simulink model "DCMotorControl_PI"  (R2024b)
settings: Solver=VariableStepAuto  StartTime=0.0  StopTime=0.2  RelTol=1e-4
InitFcn:
  | clear
  | clc
  | 
  | Power = 3336;
  | Vdc = 140;
  | Va_rated = 140;
  | Ia_rated = 25;
  | Wm_rated = 3000*2*pi/60;
  | Te_rated = Power/Wm_rated;
  | 
  | Ra = 0.26;
  | La = 1.7e-3;
  | J = 0.00252;
  | B = 0;
  | 
  | K = Te_rated/Ia_rated;
  | 
  | Wcc=500*2*pi;
  | Wcs=30*2*pi;
  | 
  | Kpc=La*Wcc;
  | Kic=Ra*Wcc;
  | Kac=1/Kpc;
  | 
  | Kps=(J*Wcs)/K;
  | Kis=(J*(Wcs)^2)/5*K;
  | Kas=1/Kps;
libraries: simulink x2
settings Model: Creator=junheehan  LastModifiedBy=junheehan

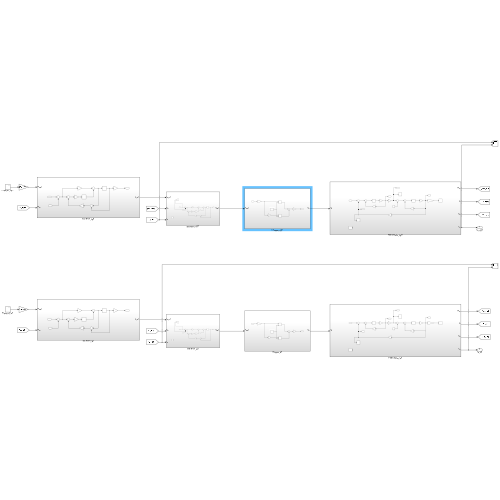
[thumbnail: Simulink's stored preview of the top-level diagram]
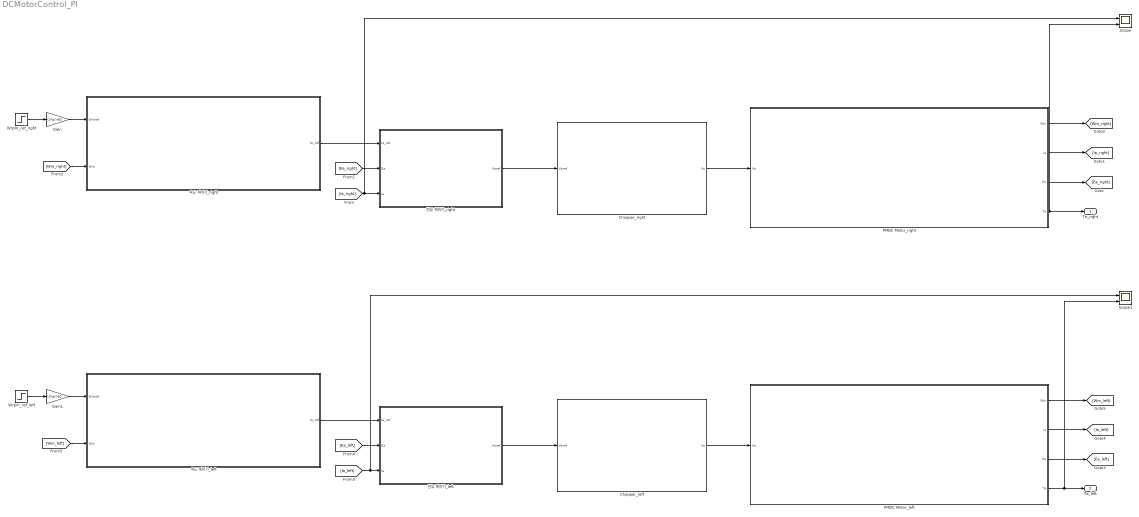
== system DCMotorControl_PI ==
  Chopper_left : Subsystem
  Chopper_right : Subsystem
  Gain : Gain  Gain=(2*pi)/60
  Gain1 : Gain  Gain=(2*pi)/60
  PMDC Motor_left : Subsystem
  PMDC Motor_right : Subsystem
  Scope : Scope  NumInputPorts=2
  Scope1 : Scope  NumInputPorts=2
  Wrpm_ref_left : Step  Time=0.05  After=2500  SampleTime=0
  Wrpm_ref_right : Step  Time=0.05  After=2500  SampleTime=0
  속도 제어기_left : Subsystem
  속도 제어기_right : Subsystem
  전류 제어기_left : Subsystem
  전류 제어기_right : Subsystem
  Te_right : Outport
  Te_left : Outport  Port=2
  wires:
  [Ea_right] -> 전류 제어기_right/2(Ea)
  [Ia_right] -> Scope/1, 전류 제어기_right/3(Ia)
  [Wm_right] -> 속도 제어기_right/2(Wm)
  속도 제어기_right/1(Ia_ref) -> 전류 제어기_right/1(Ia_ref)
  PMDC Motor_right/1(Wm) -> [Wm_right]
  PMDC Motor_right/3(Ea) -> [Ea_right]
  PMDC Motor_right/2(Ia) -> [Ia_right]
  Wrpm_ref_right/1 -> Gain/1
  Gain/1 -> 속도 제어기_right/1(Wmref)
  전류 제어기_right/1(Varef) -> Chopper_right/1(Varef)
  Chopper_right/1(Va) -> PMDC Motor_right/1(Va)
  PMDC Motor_right/4(Te) -> Scope/2, Te_right/1
  [Ea_left] -> 전류 제어기_left/2(Ea)
  전류 제어기_left/1(Varef) -> Chopper_left/1(Varef)
  PMDC Motor_left/1(Wm) -> [Wm_left]
  Gain1/1 -> 속도 제어기_left/1(Wmref)
  PMDC Motor_left/4(Te) -> Scope1/2, Te_left/1
  PMDC Motor_left/2(Ia) -> [Ia_left]
  Wrpm_ref_left/1 -> Gain1/1
  Chopper_left/1(Va) -> PMDC Motor_left/1(Va)
  [Ia_left] -> Scope1/1, 전류 제어기_left/3(Ia)
  [Wm_left] -> 속도 제어기_left/2(Wm)
  속도 제어기_left/1(Ia_ref) -> 전류 제어기_left/1(Ia_ref)
  PMDC Motor_left/3(Ea) -> [Ea_left]

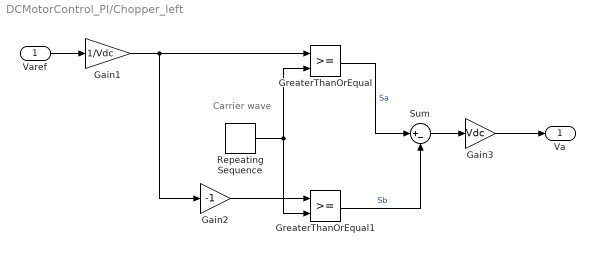
== system DCMotorControl_PI/Chopper_left ==
  note: Carrier wave
  Varef : Inport
  Gain1 : Gain  Gain=1/Vdc
  Gain2 : Gain  Gain=-1
  Gain3 : Gain  Gain=Vdc
  GreaterThanOrEqual : RelationalOperator  OutDataTypeStr=boolean  RndMeth=Simplest  InputSameDT=off
  GreaterThanOrEqual1 : RelationalOperator  OutDataTypeStr=boolean  RndMeth=Simplest  InputSameDT=off
  Repeating Sequence : simulink/Sources/Repeating Sequence  rep_seq_t=[0 1/10000 1/5000]  rep_seq_y=[-1 1 -1]
  Sum : Sum  Inputs=|+-
  Va : Outport
  wires:
  Varef/1 -> Gain1/1
  GreaterThanOrEqual1/1 -> Sum/2  "Sb"
  GreaterThanOrEqual/1 -> Sum/1  "Sa"
  Gain3/1 -> Va/1
  Repeating Sequence/1 -> GreaterThanOrEqual1/2, GreaterThanOrEqual/2
  Gain2/1 -> GreaterThanOrEqual1/1
  Gain1/1 -> Gain2/1, GreaterThanOrEqual/1
  Sum/1 -> Gain3/1

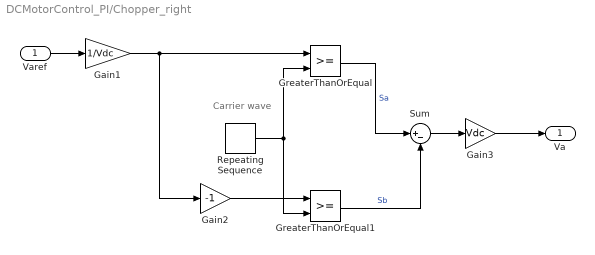
== system DCMotorControl_PI/Chopper_right ==
  note: Carrier wave
  Varef : Inport
  Gain1 : Gain  Gain=1/Vdc
  Gain2 : Gain  Gain=-1
  Gain3 : Gain  Gain=Vdc
  GreaterThanOrEqual : RelationalOperator  OutDataTypeStr=boolean  RndMeth=Simplest  InputSameDT=off
  GreaterThanOrEqual1 : RelationalOperator  OutDataTypeStr=boolean  RndMeth=Simplest  InputSameDT=off
  Repeating Sequence : simulink/Sources/Repeating Sequence  rep_seq_t=[0 1/10000 1/5000]  rep_seq_y=[-1 1 -1]
  Sum : Sum  Inputs=|+-
  Va : Outport
  wires:
  Varef/1 -> Gain1/1
  GreaterThanOrEqual1/1 -> Sum/2  "Sb"
  GreaterThanOrEqual/1 -> Sum/1  "Sa"
  Gain3/1 -> Va/1
  Repeating Sequence/1 -> GreaterThanOrEqual1/2, GreaterThanOrEqual/2
  Gain2/1 -> GreaterThanOrEqual1/1
  Gain1/1 -> Gain2/1, GreaterThanOrEqual/1
  Sum/1 -> Gain3/1

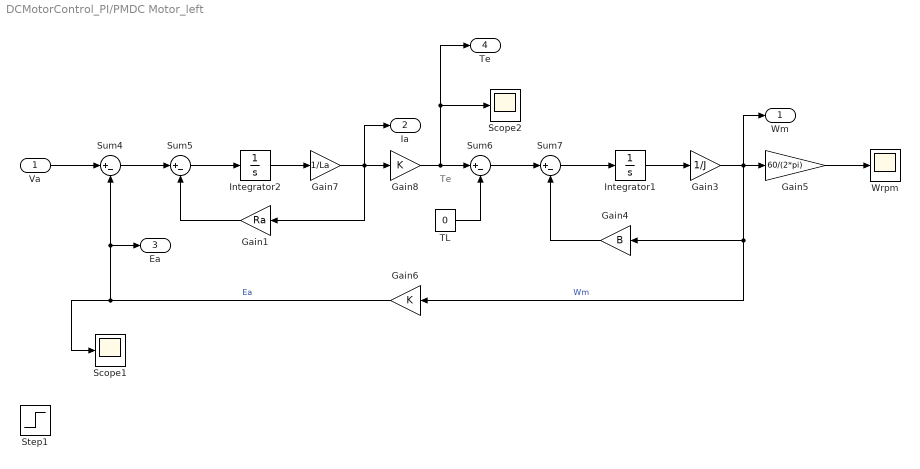
== system DCMotorControl_PI/PMDC Motor_left ==
  note: Te
  Va : Inport
  Gain1 : Gain  Gain=Ra
  Gain3 : Gain  Gain=1/J
  Gain4 : Gain  Gain=B
  Gain5 : Gain  Gain=60/(2*pi)
  Gain6 : Gain  Gain=K
  Gain7 : Gain  Gain=1/La
  Gain8 : Gain  Gain=K
  Integrator1 : Integrator
  Integrator2 : Integrator
  Scope1 : Scope
  Scope2 : Scope
  Step1 : Step  Time=0.05  After=70  SampleTime=0
  Sum{4..7} (4 alike) : Sum  Inputs=|+-
  TL : Constant  Value=0
  Wrpm : Scope
  Wm : Outport
  Ia : Outport  Port=2
  Ea : Outport  Port=3
  Te : Outport  Port=4
  wires:
  Va/1 -> Sum4/1
  Gain8/1 -> Scope2/1, Te/1, Sum6/1
  TL/1 -> Sum6/2
  Sum6/1 -> Sum7/1
  Sum4/1 -> Sum5/1
  Integrator2/1 -> Gain7/1
  Integrator1/1 -> Gain3/1
  Gain7/1 -> Gain1/1, Ia/1, Gain8/1
  Gain6/1 -> Scope1/1, Sum4/2, Ea/1  "Ea"
  Sum7/1 -> Integrator1/1
  Sum5/1 -> Integrator2/1
  Gain3/1 -> Gain6/1, Gain4/1, Wm/1, Gain5/1  "Wm"
  Gain4/1 -> Sum7/2
  Gain1/1 -> Sum5/2
  Gain5/1 -> Wrpm/1

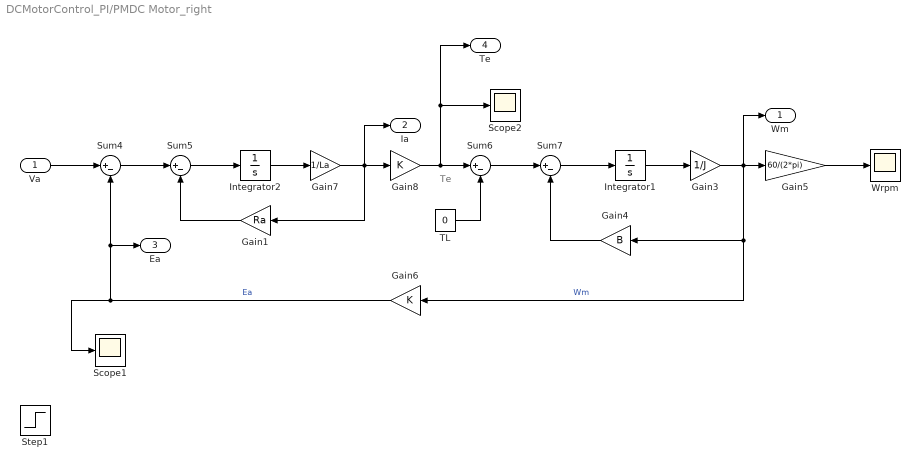
== system DCMotorControl_PI/PMDC Motor_right ==
  note: Te
  Va : Inport
  Gain1 : Gain  Gain=Ra
  Gain3 : Gain  Gain=1/J
  Gain4 : Gain  Gain=B
  Gain5 : Gain  Gain=60/(2*pi)
  Gain6 : Gain  Gain=K
  Gain7 : Gain  Gain=1/La
  Gain8 : Gain  Gain=K
  Integrator1 : Integrator
  Integrator2 : Integrator
  Scope1 : Scope
  Scope2 : Scope
  Step1 : Step  Time=0.05  After=70  SampleTime=0
  Sum{4..7} (4 alike) : Sum  Inputs=|+-
  TL : Constant  Value=0
  Wrpm : Scope
  Wm : Outport
  Ia : Outport  Port=2
  Ea : Outport  Port=3
  Te : Outport  Port=4
  wires:
  Va/1 -> Sum4/1
  Gain8/1 -> Scope2/1, Te/1, Sum6/1
  TL/1 -> Sum6/2
  Sum6/1 -> Sum7/1
  Sum4/1 -> Sum5/1
  Integrator2/1 -> Gain7/1
  Integrator1/1 -> Gain3/1
  Gain7/1 -> Gain1/1, Ia/1, Gain8/1
  Gain6/1 -> Scope1/1, Sum4/2, Ea/1  "Ea"
  Sum7/1 -> Integrator1/1
  Sum5/1 -> Integrator2/1
  Gain3/1 -> Gain6/1, Gain4/1, Wm/1, Gain5/1  "Wm"
  Gain4/1 -> Sum7/2
  Gain1/1 -> Sum5/2
  Gain5/1 -> Wrpm/1

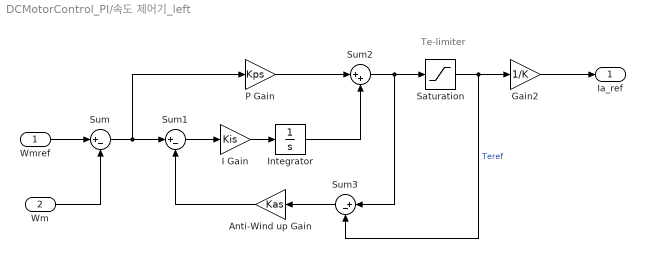
== system DCMotorControl_PI/속도 제어기_left ==
  note: Te-limiter
  Wmref : Inport
  Wm : Inport  Port=2
  Anti-Wind up Gain : Gain  Gain=Kas
  Gain2 : Gain  Gain=1/K
  I Gain : Gain  Gain=Kis
  Integrator : Integrator
  P Gain : Gain  Gain=Kps
  Saturation : Saturate  UpperLimit=Te_rated  LowerLimit=-Te_rated
  Sum : Sum  Inputs=|+-
  Sum1 : Sum  Inputs=|+-
  Sum2 : Sum  Inputs=|++
  Sum3 : Sum  Inputs=|+-
  Ia_ref : Outport
  wires:
  Wm/1 -> Sum/2
  Sum3/1 -> Anti-Wind up Gain/1
  Sum2/1 -> Saturation/1, Sum3/1
  Integrator/1 -> Sum2/2
  P Gain/1 -> Sum2/1
  Gain2/1 -> Ia_ref/1
  Anti-Wind up Gain/1 -> Sum1/2
  Sum1/1 -> I Gain/1
  I Gain/1 -> Integrator/1
  Wmref/1 -> Sum/1
  Sum/1 -> P Gain/1, Sum1/1
  Saturation/1 -> Sum3/2, Gain2/1  "Teref"

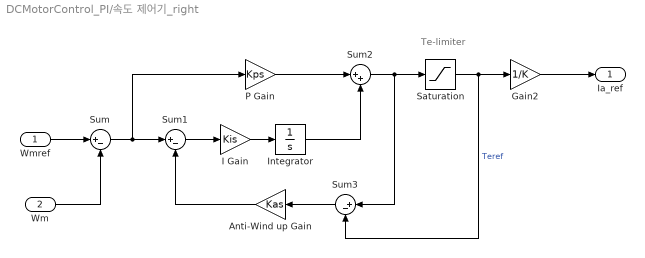
== system DCMotorControl_PI/속도 제어기_right ==
  note: Te-limiter
  Wmref : Inport
  Wm : Inport  Port=2
  Anti-Wind up Gain : Gain  Gain=Kas
  Gain2 : Gain  Gain=1/K
  I Gain : Gain  Gain=Kis
  Integrator : Integrator
  P Gain : Gain  Gain=Kps
  Saturation : Saturate  UpperLimit=Te_rated  LowerLimit=-Te_rated
  Sum : Sum  Inputs=|+-
  Sum1 : Sum  Inputs=|+-
  Sum2 : Sum  Inputs=|++
  Sum3 : Sum  Inputs=|+-
  Ia_ref : Outport
  wires:
  Wm/1 -> Sum/2
  Sum3/1 -> Anti-Wind up Gain/1
  Sum2/1 -> Saturation/1, Sum3/1
  Integrator/1 -> Sum2/2
  P Gain/1 -> Sum2/1
  Gain2/1 -> Ia_ref/1
  Anti-Wind up Gain/1 -> Sum1/2
  Sum1/1 -> I Gain/1
  I Gain/1 -> Integrator/1
  Wmref/1 -> Sum/1
  Sum/1 -> P Gain/1, Sum1/1
  Saturation/1 -> Sum3/2, Gain2/1  "Teref"

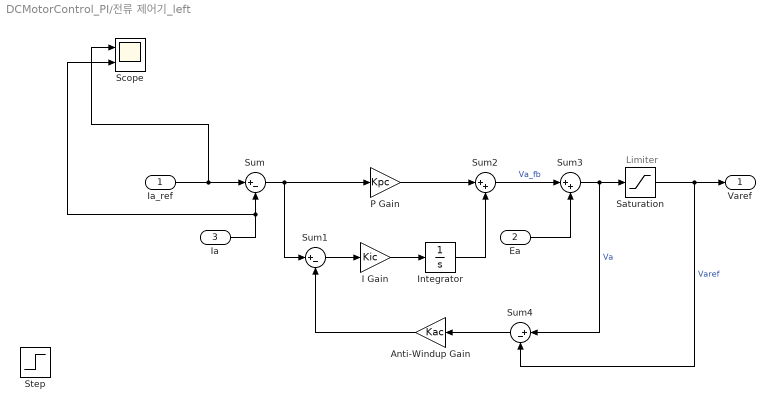
== system DCMotorControl_PI/전류 제어기_left ==
  note: Limiter
  Ia_ref : Inport
  Ea : Inport  Port=2
  Ia : Inport  Port=3
  Anti-Windup Gain : Gain  Gain=Kac
  I Gain : Gain  Gain=Kic
  Integrator : Integrator
  P Gain : Gain  Gain=Kpc
  Saturation : Saturate  UpperLimit=Va_rated  LowerLimit=-Va_rated  OutMax=[140]
  Scope : Scope  NumInputPorts=2
  Step : Step  Time=0.005  After=20  SampleTime=0
  Sum : Sum  Inputs=|+-
  Sum1 : Sum  Inputs=|+-
  Sum2 : Sum  Inputs=|++
  Sum3 : Sum  Inputs=|++
  Sum4 : Sum  Inputs=|+-
  Varef : Outport
  wires:
  Anti-Windup Gain/1 -> Sum1/2
  Ea/1 -> Sum3/2
  Sum3/1 -> Sum4/1, Saturation/1  "Va"
  I Gain/1 -> Integrator/1
  P Gain/1 -> Sum2/1
  Sum2/1 -> Sum3/1  "Va_fb"
  Integrator/1 -> Sum2/2
  Sum4/1 -> Anti-Windup Gain/1
  Saturation/1 -> Varef/1, Sum4/2  "Varef"
  Sum/1 -> Sum1/1, P Gain/1
  Sum1/1 -> I Gain/1
  Ia_ref/1 -> Scope/1, Sum/1
  Ia/1 -> Scope/2, Sum/2

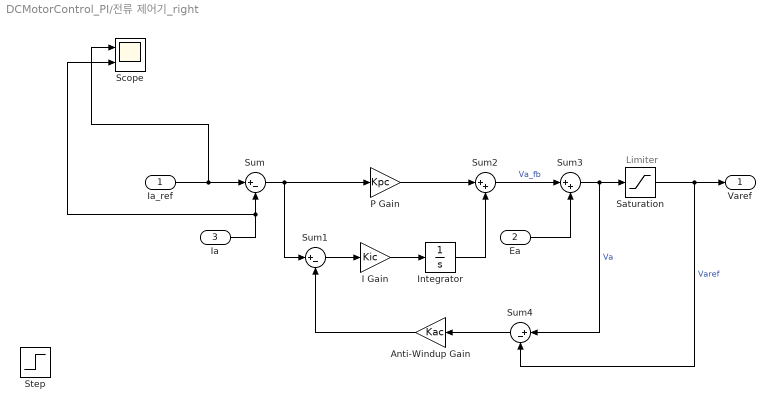
== system DCMotorControl_PI/전류 제어기_right ==
  note: Limiter
  Ia_ref : Inport
  Ea : Inport  Port=2
  Ia : Inport  Port=3
  Anti-Windup Gain : Gain  Gain=Kac
  I Gain : Gain  Gain=Kic
  Integrator : Integrator
  P Gain : Gain  Gain=Kpc
  Saturation : Saturate  UpperLimit=Va_rated  LowerLimit=-Va_rated  OutMax=[140]
  Scope : Scope  NumInputPorts=2
  Step : Step  Time=0.005  After=20  SampleTime=0
  Sum : Sum  Inputs=|+-
  Sum1 : Sum  Inputs=|+-
  Sum2 : Sum  Inputs=|++
  Sum3 : Sum  Inputs=|++
  Sum4 : Sum  Inputs=|+-
  Varef : Outport
  wires:
  Anti-Windup Gain/1 -> Sum1/2
  Ea/1 -> Sum3/2
  Sum3/1 -> Sum4/1, Saturation/1  "Va"
  I Gain/1 -> Integrator/1
  P Gain/1 -> Sum2/1
  Sum2/1 -> Sum3/1  "Va_fb"
  Integrator/1 -> Sum2/2
  Sum4/1 -> Anti-Windup Gain/1
  Saturation/1 -> Varef/1, Sum4/2  "Varef"
  Sum/1 -> Sum1/1, P Gain/1
  Sum1/1 -> I Gain/1
  Ia_ref/1 -> Scope/1, Sum/1
  Ia/1 -> Scope/2, Sum/2
